simulink model "assignment_1_c"  (R2021a)
settings: Solver=VariableStepAuto  StartTime=0.0  StopTime=10.0  RelTol=1e-3
undefined symbols (not defined in the file): c1, c2, k1, k2, m1, m2
settings Model: Creator=vedan  LastModifiedBy=vedan

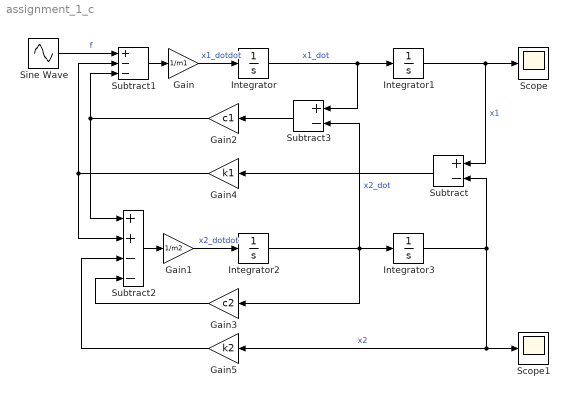
== system assignment_1_c ==
  Gain : Gain  Gain=1/m1
  Gain1 : Gain  Gain=1/m2
  Gain2 : Gain  Gain=c1
  Gain3 : Gain  Gain=c2
  Gain4 : Gain  Gain=k1
  Gain5 : Gain  Gain=k2
  Integrator{,1..3} (4 alike) : Integrator
  Scope : Scope
  Scope1 : Scope
  Sine Wave : Sin  Amplitude=3  Frequency=10  SampleTime=0
  Subtract : Sum  Inputs=+-
  Subtract1 : Sum  Inputs=+--
  Subtract2 : Sum  Inputs=++--
  Subtract3 : Sum  Inputs=+-
  wires:
  Sine Wave/1 -> Subtract1/1  "f"
  Gain5/1 -> Subtract2/3
  Gain4/1 -> Subtract1/2, Subtract2/2
  Subtract1/1 -> Gain/1
  Gain1/1 -> Integrator2/1  "x2_dotdot"
  Subtract/1 -> Gain4/1
  Gain3/1 -> Subtract2/4
  Integrator1/1 -> Scope/1, Subtract/1  "x1"
  Subtract2/1 -> Gain1/1
  Integrator3/1 -> Subtract/2, Scope1/1, Gain5/1  "x2"
  Integrator/1 -> Subtract3/1, Integrator1/1  "x1_dot"
  Gain2/1 -> Subtract1/3, Subtract2/1
  Integrator2/1 -> Subtract3/2, Gain3/1, Integrator3/1  "x2_dot"
  Subtract3/1 -> Gain2/1
  Gain/1 -> Integrator/1  "x1_dotdot"
